simulink model "dd"  (R2020a)
settings: Solver=VariableStepAuto  StartTime=0.0  StopTime=10.0  RelTol=1e-3
model workspace (MAT data in the model file):
  a = 2
  b = 2
  c = 2
settings Model: Creator=tnradm  LastModifiedBy=tnradm

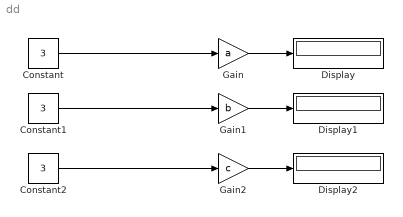
== system dd ==
  Constant : Constant  Value=3
  Constant1 : Constant  Value=3
  Constant2 : Constant  Value=3
  Display : Display
  Display1 : Display
  Display2 : Display
  Gain : Gain  Gain=a
  Gain1 : Gain  Gain=b
  Gain2 : Gain  Gain=c
  wires:
  Constant/1 -> Gain/1
  Constant1/1 -> Gain1/1
  Constant2/1 -> Gain2/1
  Gain2/1 -> Display2/1
  Gain1/1 -> Display1/1
  Gain/1 -> Display/1
